simulink model "modern_control_solve_sim"  (R2016a)
settings: Solver=FixedStepAuto  StartTime=0.0  StopTime=10.0  FixedStep=0.001  RelTol=1e-3
values from neighbouring files (symbols this model uses):
  x10 = [-2 -2 -2 -2 -2 0 1 2 2 0]    [modern_control_solve_m.m]
  x20 = [-2 -1 0 1 2 2  1  0 -2 -1]    [modern_control_solve_m.m]
settings Model: Creator=richa  LastModifiedBy=richa
settings DataIOCC: SaveFormat=Array  SaveState=on  OutputSaveName=y

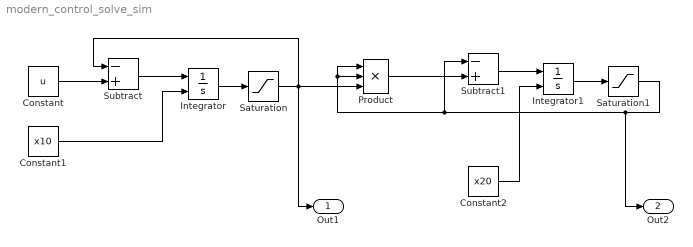
== system modern_control_solve_sim ==
  Constant : Constant  Value=u
  Constant1 : Constant  Value=x10
  Constant2 : Constant  Value=x20
  Integrator : Integrator  InitialConditionSource=external
  Integrator1 : Integrator  InitialConditionSource=external
  Product : Product  Inputs=3
  Saturation : Saturate  UpperLimit=1  LowerLimit=-1
  Saturation1 : Saturate  UpperLimit=1  LowerLimit=-1
  Subtract : Sum  Inputs=-+
  Subtract1 : Sum  Inputs=-+
  Out1 : Outport
  Out2 : Outport  Port=2
  wires:
  Constant/1 -> Subtract/2
  Subtract/1 -> Integrator/1
  Product/1 -> Subtract1/2
  Subtract1/1 -> Integrator1/1
  Constant1/1 -> Integrator/2
  Constant2/1 -> Integrator1/2
  Integrator/1 -> Saturation/1
  Saturation/1 -> Out1/1, Product/3, Subtract/1
  Integrator1/1 -> Saturation1/1
  Saturation1/1 -> Out2/1, Subtract1/1, Product/1, Product/2
